simulink library "INT_VehV_VD"  (R2016b)
settings: Solver=VariableStepAuto  StartTime=0.0  StopTime=10.0  RelTol=1e-3
settings Model: Creator=lenovo  LastModifiedBy=lenovo

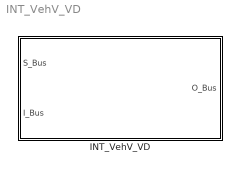
== system INT_VehV_VD ==
  INT_VehV_VD : Subsystem

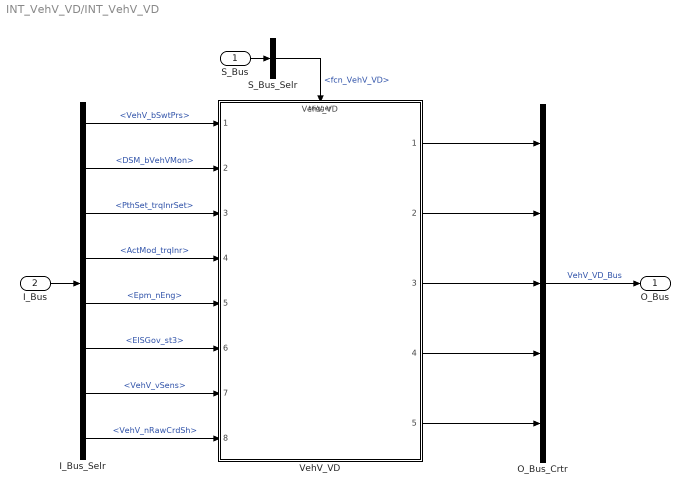
== system INT_VehV_VD/INT_VehV_VD ==
  S_Bus : Inport
  I_Bus : Inport  Port=2
  I_Bus_Selr : BusSelector  OutputSignals=VehV_bSwtPrs,DSM_bVehVMon,PthSet_trqInrSet,ActMod_trqInr,Epm_nEng,EISGov_st3,VehV_vSens,VehV_nRawCrdSh
  O_Bus_Crtr : BusCreator  Inputs=5
  S_Bus_Selr : BusSelector  OutputSignals=fcn_VehV_VD
  VehV_VD : ModelReference  ModelNameDialog=VehV_VD  SimulationMode=Normal  ModelReferenceVersion=1.8  TriggerPortName=function  TriggerPortTriggerType=function-call  TriggerPortStatesWhenEnabling=held
  O_Bus : Outport
  wires:
  S_Bus_Selr/1 -> VehV_VD/Trigger  "<fcn_VehV_VD>"
  S_Bus/1 -> S_Bus_Selr/1
  I_Bus/1 -> I_Bus_Selr/1
  I_Bus_Selr/1 -> VehV_VD/1  "<VehV_bSwtPrs>"
  I_Bus_Selr/2 -> VehV_VD/2  "<DSM_bVehVMon>"
  I_Bus_Selr/3 -> VehV_VD/3  "<PthSet_trqInrSet>"
  I_Bus_Selr/4 -> VehV_VD/4  "<ActMod_trqInr>"
  I_Bus_Selr/5 -> VehV_VD/5  "<Epm_nEng>"
  I_Bus_Selr/6 -> VehV_VD/6  "<EISGov_st3>"
  I_Bus_Selr/7 -> VehV_VD/7  "<VehV_vSens>"
  I_Bus_Selr/8 -> VehV_VD/8  "<VehV_nRawCrdSh>"
  O_Bus_Crtr/1 -> O_Bus/1  "VehV_VD_Bus"
  VehV_VD/1 -> O_Bus_Crtr/1
  VehV_VD/2 -> O_Bus_Crtr/2
  VehV_VD/3 -> O_Bus_Crtr/3
  VehV_VD/4 -> O_Bus_Crtr/4
  VehV_VD/5 -> O_Bus_Crtr/5
